simulink model "demo6"  (Simulink 4.00)
settings: Solver=ode45  StartTime=0.0  StopTime=20.0  RelTol=1e-3
undefined symbols (not defined in the file or in its folder): cond, gcamera, visjac
libraries: roblocks x4, simulink3 x1
settings Model: Creator=pic  LastModifiedBy=pic  LimitDataPoints=off  ExtModeTrigMode=oneshot  ExtModeArmWhenConnect=off  BlockReductionOpt=off

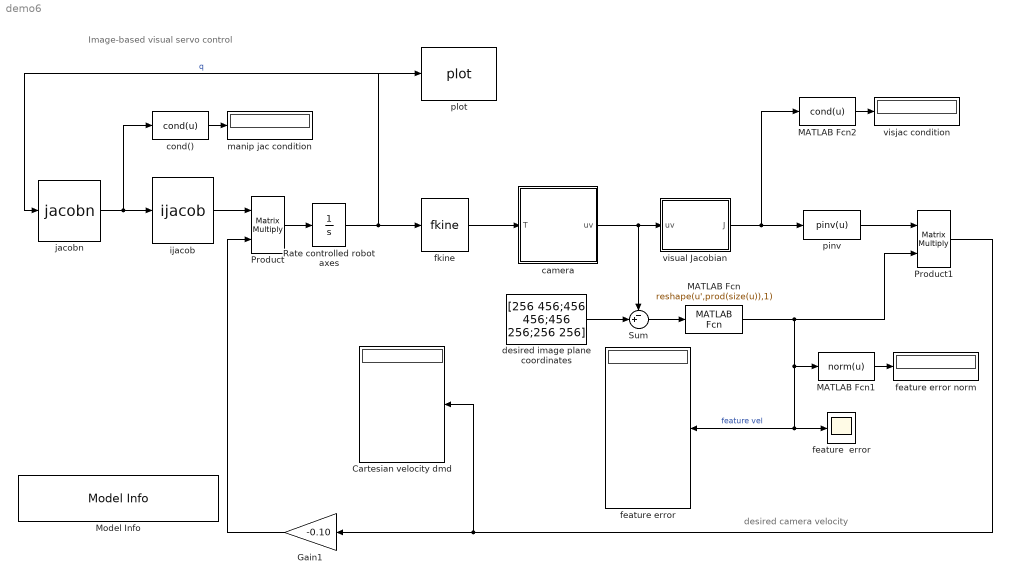
== system demo6 ==
  note: Image-based visual servo control
  note: desired camera velocity
  Cartesian velocity dmd : Display
      settings: Format=bank
  Gain1 : Gain  Orientation=left  Gain=-0.10  Multiplication=Element-wise(K.*u)  SaturateOnIntegerOverflow=on
  MATLAB Fcn : MATLABFcn  MATLABFcn=reshape(u',prod(size(u)),1)  OutputDimensions=-1  OutputSignalType=auto  Output1D=on
  MATLAB Fcn1 : MATLABFcn  MATLABFcn=norm(u)  OutputDimensions=-1  OutputSignalType=auto  Output1D=on
  MATLAB Fcn2 : MATLABFcn  MATLABFcn=cond(u)  OutputDimensions=-1  OutputSignalType=auto  Output1D=on
  Model Info : simulink3/Signals & Systems/Model Info  InitialBlockCM=none  BlockCM=none  Frame=on  DisplayStringWithTags=|  HorizontalTextAlignment=Left  LeftAlignmentValue=0.02  SourceBlockDiagram=demo6  TagMaxNumber=20
      | Image-based visual servo control
      | %<Creator>
      | %<LastModificationDate>
  Product : Product  Inputs=2  Multiplication=Matrix(*)  SaturateOnIntegerOverflow=on
  Product1 : Product  Inputs=2  Multiplication=Matrix(*)  SaturateOnIntegerOverflow=on
  Rate controlled robot axes : Integrator  ExternalReset=none  InitialConditionSource=internal  InitialCondition="[0.3048   -0.9869    0.4483   -0.3513   -1.0595    0.1774]"  LimitOutput=off  UpperSaturationLimit=inf  LowerSaturationLimit=-inf  ShowSaturationPort=off  ShowStatePort=off  AbsoluteTolerance=auto
  Sum : Sum  Inputs=-+|  SaturateOnIntegerOverflow=on
  camera : Subsystem  mask{name=IBVS camera, camdata=[8e-3 80e3 80e3 256 256], dims=[0 511 0 511], points=rotz(0.02)*[2 0.2 0.2;2 0.2 -0.2; 2 -0.2 -0.2 ;2 -0.2 0.2]}
      mask prompts: camdata "Camera params"; dims "Image plane size"; points "Points (nx2)"
      mask init:
      | h=gcamera(name,camcalp_c(camdata),dims);
      settings: RTWFcnNameOpts=Auto  RTWFileNameOpts=Auto
  cond() : MATLABFcn  MATLABFcn=cond(u)  OutputDimensions=-1  OutputSignalType=auto  Output1D=on
  desired image plane coordinates : Constant  Value=[256 456;456 456;456 256;256 256]  VectorParams1D=off
  feature  error : Scope
      settings: TimeRange=20  YMin=-0.2  YMax=0.1  SaveToWorkspace=off  SaveName=ScopeData  LimitDataPoints=on  MaxDataPoints=5000
  feature error : Display
      settings: Format=bank
  feature error norm : Display
      settings: Format=short
  fkine : roblocks/fkine  robot=p560
  ijacob : roblocks/ijacob
  jacobn : roblocks/jacobn  robot=p560
  manip jac condition : Display
      settings: Format=short
  pinv : MATLABFcn  MATLABFcn=pinv(u)  OutputDimensions=-1  OutputSignalType=auto  Output1D=off
  plot : roblocks/plot  robot=p560
  visjac condition : Display
      settings: Format=short
  visual Jacobian : Subsystem  mask{camdata=[8e-3 80e3 80e3 256 256], z=2}
      mask prompts: camdata "Camera params"; z "Assumed depth (m)"
      settings: RTWFcnNameOpts=Auto  RTWFileNameOpts=Auto
  wires:
  Rate controlled robot axes/1 -> fkine/1, plot/1, jacobn/1  "q"
  jacobn/1 -> ijacob/1, cond()/1
  Product/1 -> Rate controlled robot axes/1
  camera/1(uv) -> visual Jacobian/1(uv), Sum/1
  fkine/1 -> camera/1(T)
  visual Jacobian/1(J) -> pinv/1, MATLAB Fcn2/1
  Sum/1 -> MATLAB Fcn/1
  pinv/1 -> Product1/1
  desired image plane coordinates/1 -> Sum/2
  MATLAB Fcn/1 -> Product1/2, MATLAB Fcn1/1, feature error/1, feature  error/1  "feature vel"
  ijacob/1 -> Product/1
  MATLAB Fcn2/1 -> visjac condition/1
  cond()/1 -> manip jac condition/1
  MATLAB Fcn1/1 -> feature error norm/1
  Product1/1 -> Gain1/1, Cartesian velocity dmd/1
  Gain1/1 -> Product/2

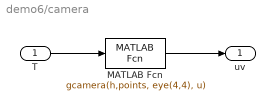
== system demo6/camera ==
  T : Inport  Port=1
  MATLAB Fcn : MATLABFcn  MATLABFcn=gcamera(h,points, eye(4,4), u)  OutputDimensions=-1  OutputSignalType=auto  Output1D=off
  uv : Outport  Port=1
  wires:
  MATLAB Fcn/1 -> uv/1
  T/1 -> MATLAB Fcn/1

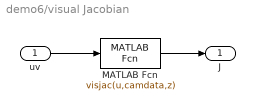
== system demo6/visual Jacobian ==
  uv : Inport  Port=1
  MATLAB Fcn : MATLABFcn  MATLABFcn=visjac(u,camdata,z)  OutputDimensions=[8 6]  OutputSignalType=auto  Output1D=off
  J : Outport  Port=1
  wires:
  MATLAB Fcn/1 -> J/1
  uv/1 -> MATLAB Fcn/1
